simulink model "CSTR_sim"  (R2022b)
settings: Solver=ode8  StartTime=0.0  StopTime=t_end  FixedStep=Ts  RelTol=1e-3
undefined symbols (not defined in the file): A, B, C, Ca, Cb, Fa0, Fb0, kv, kw, tFa_down, tFa_up, tFb_down, tFb_up, V, xa0, y
settings Model: Creator=Ivona  LastModifiedBy=Milosh Yokich
settings SolverCC: AlgebraicLoopSolver=TrustRegion
settings DataIOCC: ReturnWorkspaceOutputs=off
settings DebuggingCC: UnconnectedInputMsg=warning  UnconnectedOutputMsg=warning  UnconnectedLineMsg=warning  SFMachineParentedDataDiag=warning  ArithmeticOperatorsInVariantConditions=warning
settings ModelReferenceCC: EnableRefExpFcnMdlSchedulingChecks=on
settings SFSimCC: SimUseLocalCustomCode=off  CustomCodeUndefinedFunction=UseInterfaceOnly
settings RTWCC: RTWUseLocalCustomCode=off
settings CodeAppCC: StateflowObjectComments=on
settings SimscapeCC: SimscapeNormalizeSystem=off

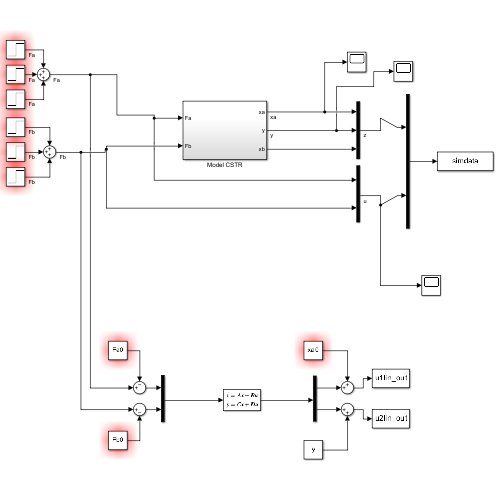
[thumbnail: Simulink's stored preview of the top-level diagram]
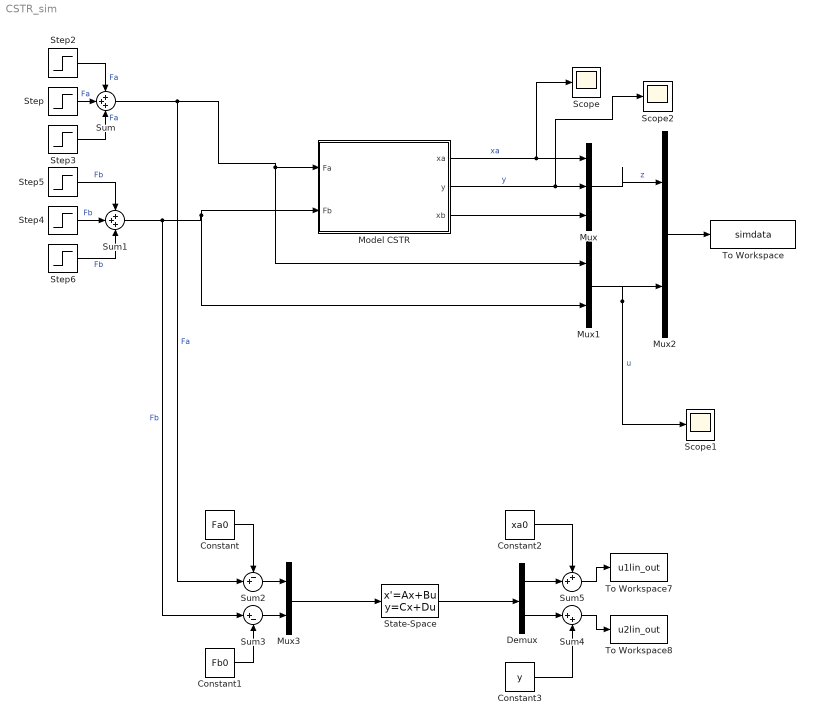
== system CSTR_sim ==
  Constant : Constant  Value=Fa0
  Constant1 : Constant  Value=Fb0
  Constant2 : Constant  Value=xa0
  Constant3 : Constant  Value=y
  Demux : Demux  Outputs=2
  Model CSTR : Subsystem
  Mux : Mux  Inputs=3
  Mux1 : Mux  Inputs=2
  Mux2 : Mux  Inputs=2
  Mux3 : Mux  Inputs=2
  Scope : Scope
  Scope1 : Scope
  Scope2 : Scope
  State-Space : StateSpace  A=A  B=B  C=C  D=[0 0;0 0]  InitialCondition=0
  Step : Step  Time=0  After=Fa0  SampleTime=0
  Step2 : Step  Time=tFa_up  After=0.1*Fa0  SampleTime=0
  Step3 : Step  Time=tFa_down  After=-0.1*Fa0  SampleTime=0
  Step4 : Step  Time=0  After=Fb0  SampleTime=0
  Step5 : Step  Time=tFb_up  After=0.1*Fb0  SampleTime=0
  Step6 : Step  Time=tFb_down  After=-0.1*Fb0  SampleTime=0
  Sum : Sum  Inputs=+++
  Sum1 : Sum  Inputs=+++
  Sum2 : Sum  Inputs=-+|
  Sum3 : Sum  Inputs=|+-
  Sum4 : Sum  Inputs=|++
  Sum5 : Sum  Inputs=++|
  To Workspace : ToWorkspace  VariableName=simdata  SaveFormat=Timeseries  SampleTime=-1
  To Workspace7 : ToWorkspace  VariableName=u1lin_out  SampleTime=-1
  To Workspace8 : ToWorkspace  VariableName=u2lin_out  SampleTime=-1
  wires:
  Model CSTR/1(xa) -> Mux/1, Scope/1  "xa"
  Model CSTR/2(y) -> Mux/2, Scope2/1  "y"
  Mux/1 -> Mux2/1  "z"
  Mux1/1 -> Scope1/1, Mux2/2  "u"
  Mux2/1 -> To Workspace/1
  Step/1 -> Sum/2  "Fa"
  Step2/1 -> Sum/1  "Fa"
  Step3/1 -> Sum/3  "Fa"
  Sum/1 -> Sum2/2, Mux1/1, Model CSTR/1(Fa)  "Fa"
  Step4/1 -> Sum1/2  "Fb"
  Step6/1 -> Sum1/3  "Fb"
  Step5/1 -> Sum1/1  "Fb"
  Sum1/1 -> Sum3/1, Mux1/2, Model CSTR/2(Fb)  "Fb"
  Model CSTR/3(xb) -> Mux/3
  Sum4/1 -> To Workspace8/1
  Constant2/1 -> Sum5/1
  Constant3/1 -> Sum4/2
  Constant1/1 -> Sum3/2
  Sum5/1 -> To Workspace7/1
  Constant/1 -> Sum2/1
  State-Space/1 -> Demux/1
  Demux/2 -> Sum4/1
  Sum2/1 -> Mux3/1
  Demux/1 -> Sum5/2
  Sum3/1 -> Mux3/2
  Mux3/1 -> State-Space/1

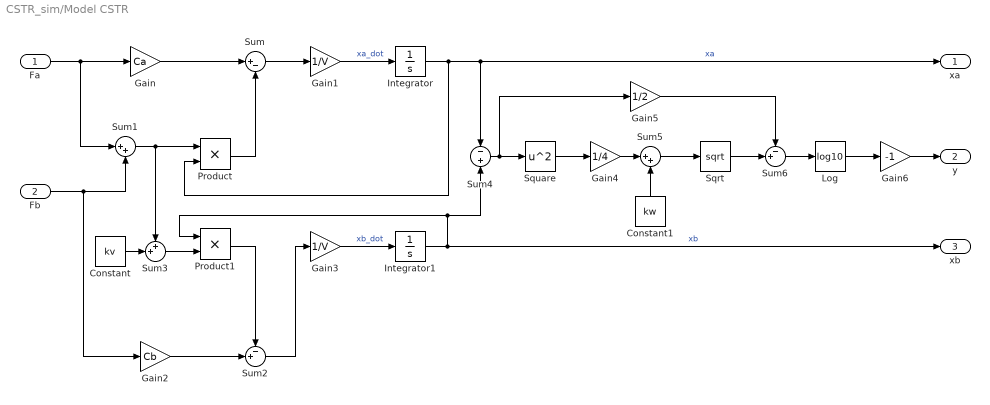
== system CSTR_sim/Model CSTR ==
  Fa : Inport
  Fb : Inport  Port=2
  Constant : Constant  Value=kv
  Constant1 : Constant  Value=kw
  Gain : Gain  Gain=Ca
  Gain1 : Gain  Gain=1/V
  Gain2 : Gain  Gain=Cb
  Gain3 : Gain  Gain=1/V
  Gain4 : Gain  Gain=1/4
  Gain5 : Gain  Gain=1/2
  Gain6 : Gain  Gain=-1
  Integrator : Integrator
  Integrator1 : Integrator
  Log : Math  Operator=log10  SignedPower=on
  Product : Product
  Product1 : Product
  Sqrt : Sqrt
  Square : Math  Operator=square  SignedPower=on
  Sum : Sum  Inputs=|+-
  Sum1 : Sum  Inputs=|++
  Sum2 : Sum  Inputs=-+|
  Sum3 : Sum  Inputs=++|
  Sum4 : Sum  Inputs=-+
  Sum5 : Sum  Inputs=|++
  Sum6 : Sum  Inputs=-+|
  xa : Outport
  y : Outport  Port=2
  xb : Outport  Port=3
  wires:
  Integrator/1 -> Product/2, Sum4/1, xa/1  "xa"
  Fa/1 -> Sum1/1, Gain/1
  Gain/1 -> Sum/1
  Fb/1 -> Gain2/1, Sum1/2
  Sum1/1 -> Sum3/1, Product/1
  Product/1 -> Sum/2
  Sum/1 -> Gain1/1
  Gain1/1 -> Integrator/1  "xa_dot"
  Gain2/1 -> Sum2/2
  Constant/1 -> Sum3/2
  Product1/1 -> Sum2/1
  Sum2/1 -> Gain3/1
  Integrator1/1 -> xb/1, Sum4/2, Product1/1  "xb"
  Sum3/1 -> Product1/2
  Gain3/1 -> Integrator1/1  "xb_dot"
  Square/1 -> Gain4/1
  Gain4/1 -> Sum5/1
  Constant1/1 -> Sum5/2
  Sum5/1 -> Sqrt/1
  Sqrt/1 -> Sum6/2
  Gain5/1 -> Sum6/1
  Sum6/1 -> Log/1
  Log/1 -> Gain6/1
  Gain6/1 -> y/1
  Sum4/1 -> Gain5/1, Square/1
